simulink model "dcac_averaged"  (Simulink 6.5)
settings: Solver=ode45  StartTime=0.0  StopTime=1/60  MaxStep=0.1e-3  RelTol=1e-3
settings Model: Creator=Mama  LastModifiedBy=Dragan Maksimovic
settings DebuggingCC: AlgebraicLoopMsg=none  SolverPrmCheckMsg=none  UnconnectedOutputMsg=none

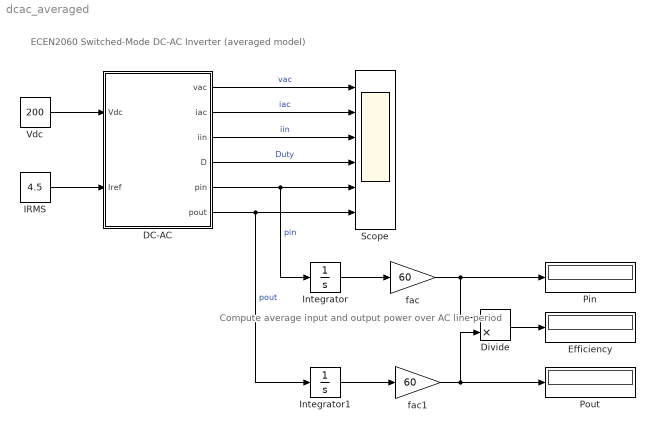
== system dcac_averaged ==
  note: ECEN2060
      | Switched-Mode DC-AC Inverter (averaged model)
  note: Compute average input and
      | output power over AC line period
  DC-AC : Subsystem  mask{Vrms=120, f=60, RL=0.8, IQ=0.05}
      mask prompts: Vrms "AC line RMS voltage"; f "AC line frequency"; RL "Output port series resistance"; IQ "Switching loss current"
      mask help: Averaged model of a switched-mode DC-AC inverter for single-phase grid-connected systems. Output ac current is in phase with the output ac line voltage, and has RMS value set by the reference input. Conduction losses are modeled by a series resistor RL at the output. Switching and other losses are modeled by a current source Isw in parallel with the DC input voltage.
      mask Display:
      | text(0.5,0.75,'DC-AC','horizontalAlignment', 'center');
      | text(0.5,0.6,'inverter','horizontalAlignment', 'center');
      | text(0.5,0.45,'(averaged)','horizontalAlignment', 'center');
  Divide : Product  Inputs=/*  OutScaling=2^-10
  Efficiency : Display
  IRMS : Constant  Value=4.5  OutDataType=sfix(16)  ConRadixGroup=Use specified scaling  OutScaling=2^0  SampleTime=inf  FramePeriod=inf
  Integrator : Integrator
  Integrator1 : Integrator
  Pin : Display
  Pout : Display
  Scope : Scope  NumInputPorts=6
      settings: TimeRange=0.018  YMin=-200~-10~0~0~0~0  YMax=200~10~8~1~1500~1500
  Vdc : Constant  Value=200  OutDataType=sfix(16)  ConRadixGroup=Use specified scaling  OutScaling=2^0  SampleTime=inf  FramePeriod=inf
  fac : Gain  Gain=60
  fac1 : Gain  Gain=60
  wires:
  Vdc/1 -> DC-AC/1(Vdc)
  IRMS/1 -> DC-AC/2(Iref)
  DC-AC/1(vac) -> Scope/1  "vac"
  DC-AC/2(iac) -> Scope/2  "iac"
  DC-AC/3(iin) -> Scope/3  "iin"
  DC-AC/4(D) -> Scope/4  "Duty"
  DC-AC/5(pin) -> Scope/5, Integrator/1  "pin"
  DC-AC/6(pout) -> Scope/6, Integrator1/1  "pout"
  Integrator/1 -> fac/1
  Integrator1/1 -> fac1/1
  Divide/1 -> Efficiency/1
  fac/1 -> Pin/1, Divide/1
  fac1/1 -> Pout/1, Divide/2

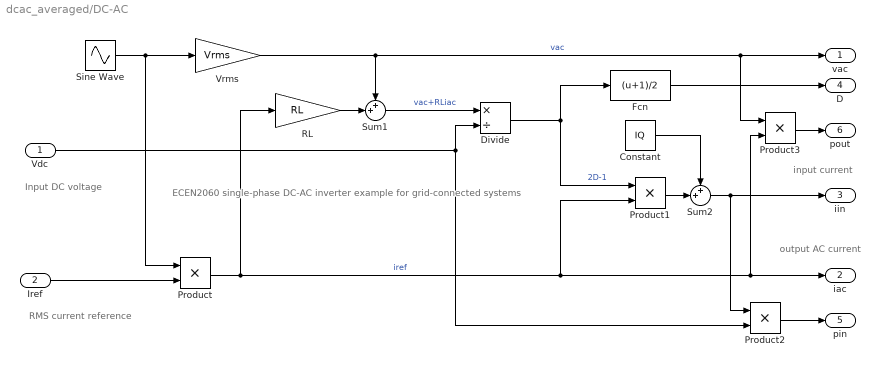
== system dcac_averaged/DC-AC ==
  note: output AC current
  note: Input DC voltage
  note: RMS current reference
  note: input current
  note: ECEN2060
      | single-phase DC-AC inverter example
      | for grid-connected systems
  Vdc : Inport
  Iref : Inport  Port=2
  Constant : Constant  Value=IQ  OutDataType=sfix(16)  ConRadixGroup=Use specified scaling  OutScaling=2^0  SampleTime=inf  FramePeriod=inf
  Divide : Product  Inputs=*/  OutScaling=2^-10
  Fcn : Fcn  Expr=(u+1)/2
  Product{,1..3} (4 alike) : Product  RndMeth=Zero
  RL : Gain  Gain=RL
  Sine Wave : Sin  Amplitude=1*sqrt(2)  Frequency=2*pi*f  SampleTime=0
  Sum1 : Sum  Inputs=++|
  Sum2 : Sum  Inputs=++|
  Vrms : Gain  Gain=Vrms
  vac : Outport
  iac : Outport  Port=2
  iin : Outport  Port=3
  D : Outport  Port=4
  pin : Outport  Port=5
  pout : Outport  Port=6
  wires:
  Sine Wave/1 -> Vrms/1, Product/1
  Vrms/1 -> Sum1/1, vac/1, Product3/1  "vac"
  Product/1 -> RL/1, Product1/2, iac/1, Product3/2  "iref"
  Iref/1 -> Product/2
  RL/1 -> Sum1/2
  Sum1/1 -> Divide/1  "vac+RLiac"
  Vdc/1 -> Divide/2, Product2/2
  Divide/1 -> Product1/1, Fcn/1  "2D-1"
  Product1/1 -> Sum2/2
  Constant/1 -> Sum2/1
  Sum2/1 -> Product2/1, iin/1
  Fcn/1 -> D/1
  Product2/1 -> pin/1
  Product3/1 -> pout/1
